simulink model "Rearranged_With_Subsystems"  (R2022b)
settings: Solver=ode15s  StartTime=0.0  StopTime=400  RelTol=1e-3
InitFcn:
  | ManipulatorSetup
  | init_quad_new_leg_raibert_strategy_v2
values from neighbouring files (symbols this model uses):
  body = 'obstacle'+string(i)    [GUIWithNavigation.m]    (also in RunModel.m)
  endx = 18    [EnvironmentData.mat]    (also in Practice data.mat = 15)
  endy = 18    [EnvironmentData.mat]    (also in Practice data.mat = 14)
  floorl = 20    [EnvironmentData.mat]    (also in GUIWithNavigation.m; Practice data.mat; RunModel.m)
  floorw = 20    [EnvironmentData.mat]    (also in GUIWithNavigation.m; Practice data.mat; RunModel.m)
  planner = plannerRRTStar(ss,stateValidator)    [GUIWithNavigation.m]    (also in RunModel.m)
  startx = 3    [EnvironmentData.mat]    (also in Practice data.mat = 2)
  starty = 3    [EnvironmentData.mat]    (also in Practice data.mat = 2)
  tar1Len = 10    [EnvironmentData.mat]    (also in GUIWithNavigation.m = length(target1); Practice data.mat = 13; RunModel.m = length(target1))
  target = [3 4.99844642156 6.95141646815 8.78790598722 9.67257563911 9.70990834754 10.5092252376 9.30187214417 9.05327436398 9.4 9.4 10.8486938703 ... (44 elements, 22x2)]    [EnvironmentData.mat]    (also in GUIWithNavigation.m = cat(1,target1,target2); Practice data.mat = [2 3.44057581018 5.07942513831 5.42542290116 7.21306818311 8; RunModel.m = cat(1,target1,target2))
  tarLen = 22    [EnvironmentData.mat]    (also in RunModel.m = length(target))
undefined symbols (not defined in the file or in its folder): closeFingers, ctrl, Extr_Data_LinkEndHole, grabObjectAngles, grabObjectAngles2, ground, holdFingers, homeAngles, inverseKinematicWeights, l1, l2, m1, m2, openFingers, readyAngles, X, Y, Z
libraries: sm_lib x459, nesl_utility x134, slpidlib x31, fl_ps_legacy_lib x6, robotmaniplib x6, simulink x5, fl_lib x5, Contact_Forces_Lib x4, Parts_Lib x4, sharedtransform x2, dspstat3 x1
(part 1 of 16)
settings Model: Creator=biorobotics  LastModifiedBy=uos
settings SolverCC: ZeroCrossAlgorithm=Adaptive  AlgebraicLoopSolver=TrustRegion
settings DataIOCC: ReturnWorkspaceOutputs=off
settings DebuggingCC: IgnoredZcDiagnostic=none  UnconnectedInputMsg=warning  UnconnectedOutputMsg=warning  UnconnectedLineMsg=warning  SFMachineParentedDataDiag=warning  ArithmeticOperatorsInVariantConditions=warning
settings ModelReferenceCC: EnableRefExpFcnMdlSchedulingChecks=on
settings SFSimCC: SimUseLocalCustomCode=off  CustomCodeUndefinedFunction=UseInterfaceOnly
settings RTWCC: RTWUseLocalCustomCode=off
settings DiagnosticsConfigSet: SimMechanicsRigidlyBoundBlock=none

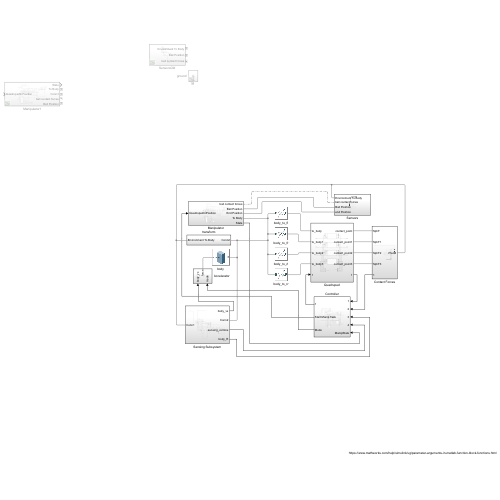
[thumbnail: Simulink's stored preview of the top-level diagram]
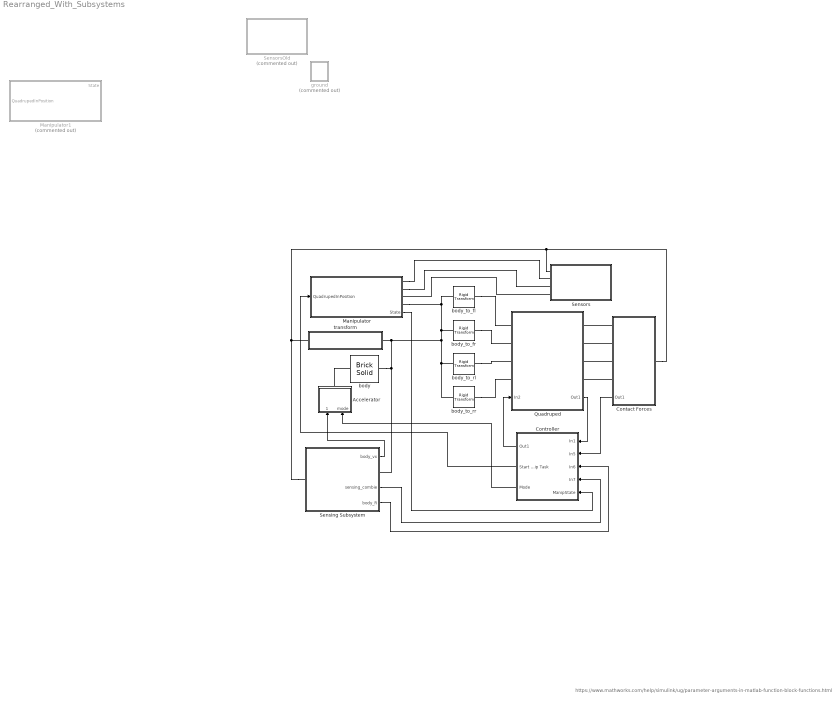
== system Rearranged_With_Subsystems ==
  note: https://www.mathworks.com/help/simulink/ug/parameter-arguments-in-matlab-function-block-functions.html
  Accelerator : Subsystem
      settings: PortSchema="{\"entries\":[{\"content\":{\"sides\":[{\"content\":{\"connectorIds\":[]},\"type\":\"ConnectorPlacement.EquallySpacedRectSide\",\"uuid\":\"3b8f4fb7-757d-44b0-8c84-ca404449afa6\"},{\"content\":{\"connectorIds\":[],\"side\":\"RIGHT\"},\"type\":\"ConnectorPlacement.EquallySpacedRectSide\",\"uuid\":\"4616ca68-8bb0-4699-a428-07415450d0e5\"},{\"content\":{\"connectorIds\":[\"LConn1\"],\"side\":\"TOP\"},\"type\":\"ConnectorPlacement.EquallySpacedRectSide\",\"uuid\":\"645a5e81-e5eb-476d-aa61-d9d757a3e189\"},{\"content\":{\"connectorIds\":[\"In1\",\"In2\"],\"side\":\"BOTTOM\"},\"type\":\"ConnectorPlacement.EquallySpacedRectSide\",\"uuid\":\"cfb89a5a-1661-4756-b538-cb5bbef02c9e\"}]},\"type\":\"ConnectorPlacement.EquallySpacedConnector\",\"uuid\":\"e64cce85-18e1-40ef-8b4c-1f7664925565\"}],\"packageUris\":[\"http://schema.mathworks.com/mf0/Connector/R2020b\"],\"version\":\"1.0\"}"
  Contact Forces : Subsystem
      settings: PortSchema="{\"entries\":[{\"content\":{\"sides\":[{\"content\":{\"connectorIds\":[\"LConn1\"]},\"type\":\"ConnectorPlacement.EquallySpacedRectSide\",\"uuid\":\"d9e77396-55f4-49e5-9c59-62df65a9aa33\"},{\"content\":{\"connectorIds\":[\"RConn1\",\"RConn2\",\"RConn3\",\"RConn4\",\"Out1\"],\"side\":\"RIGHT\"},\"type\":\"ConnectorPlacement.EquallySpacedRectSide\",\"uuid\":\"d655d73a-1d80-4dc0-89ee-c033d671b0c2\"},{\"content\":{\"connectorIds\":[],\"side\":\"TOP\"},\"type\":\"ConnectorPlacement.EquallySpacedRectSide\",\"uuid\":\"dc54e94d-e523-4784-8fd3-8e1e99781185\"},{\"content\":{\"connectorIds\":[],\"side\":\"BOTTOM\"},\"type\":\"ConnectorPlacement.EquallySpacedRectSide\",\"uuid\":\"f3bba4af-9235-4cb2-90c5-839fa8331c16\"}]},\"type\":\"ConnectorPlacement.EquallySpacedConnector\",\"uuid\":\"27dcd2a5-23bc-405e-9f4b-2eee189b7bee\"}],\"packageUris\":[\"http://schema.mathworks.com/mf0/Connector/R2020b\"],\"version\":\"1.0\"}"
  Controller : Subsystem
  Manipulator : Subsystem
      settings: PortSchema="{\"entries\":[{\"content\":{\"sides\":[{\"content\":{\"connectorIds\":[\"In1\"]},\"type\":\"ConnectorPlacement.EquallySpacedRectSide\",\"uuid\":\"ff2767ab-448c-4c0d-a9a4-8f0f2a440df5\"},{\"content\":{\"connectorIds\":[\"RConn1\",\"RConn2\",\"RConn3\",\"RConn4\",\"Out1\"],\"side\":\"RIGHT\"},\"type\":\"ConnectorPlacement.EquallySpacedRectSide\",\"uuid\":\"93606e9f-72dd-49b1-b6cf-e4d0c20d1a1a\"},{\"content\":{\"connectorIds\":[],\"side\":\"TOP\"},\"type\":\"ConnectorPlacement.EquallySpacedRectSide\",\"uuid\":\"db3624f7-6a1f-43d3-93ac-44b301eed69d\"}]},\"type\":\"ConnectorPlacement.EquallySpacedConnector\",\"uuid\":\"db27b8b3-f381-4b8d-9dee-3bd6b54b8be1\"}],\"packageUris\":[\"http://schema.mathworks.com/mf0/Connector/R2020b\"],\"version\":\"1.0\"}"
  Manipulator1 : Subsystem  Commented=on
  Quadruped : Subsystem
      settings: PortSchema="{\"entries\":[{\"content\":{\"sides\":[{\"content\":{\"connectorIds\":[\"LConn1\",\"LConn2\",\"LConn3\",\"LConn4\",\"In1\"]},\"type\":\"ConnectorPlacement.EquallySpacedRectSide\",\"uuid\":\"2b490502-7c0f-46f9-b6ce-17355d87bc82\"},{\"content\":{\"connectorIds\":[\"RConn1\",\"RConn2\",\"RConn3\",\"RConn4\",\"Out1\"],\"side\":\"RIGHT\"},\"type\":\"ConnectorPlacement.EquallySpacedRectSide\",\"uuid\":\"dcbb9991-2202-44f3-91f9-18bd7c5b50b3\"},{\"content\":{\"connectorIds\":[],\"side\":\"TOP\"},\"type\":\"ConnectorPlacement.EquallySpacedRectSide\",\"uuid\":\"5cc15507-c434-473a-bef2-323e772bf8f9\"}]},\"type\":\"ConnectorPlacement.EquallySpacedConnector\",\"uuid\":\"8c4551e2-5a1d-42e3-907a-2af9d6bfb3ed\"}],\"packageUris\":[\"http://schema.mathworks.com/mf0/Connector/R2020b\"],\"version\":\"1.0\"}"
  "Sensing Subsystem " : Subsystem
      settings: PortSchema="{\"entries\":[{\"content\":{\"sides\":[{\"content\":{\"connectorIds\":[\"LConn1\"]},\"type\":\"ConnectorPlacement.EquallySpacedRectSide\",\"uuid\":\"998221ad-fab7-44d6-86a8-33fec3ebf2d5\"},{\"content\":{\"connectorIds\":[\"Out1\",\"RConn1\",\"Out2\",\"Out3\"],\"side\":\"RIGHT\"},\"type\":\"ConnectorPlacement.EquallySpacedRectSide\",\"uuid\":\"413d99db-2567-4cd5-a930-0d9916e7d919\"},{\"content\":{\"connectorIds\":[],\"side\":\"TOP\"},\"type\":\"ConnectorPlacement.EquallySpacedRectSide\",\"uuid\":\"948855a1-4bad-45fb-bb01-4a3cbeb58f0f\"}]},\"type\":\"ConnectorPlacement.EquallySpacedConnector\",\"uuid\":\"705e2a16-9022-494f-aa05-78e7d130aa9c\"}],\"packageUris\":[\"http://schema.mathworks.com/mf0/Connector/R2020b\"],\"version\":\"1.0\"}"
  Sensors : Subsystem
  SensorsOld : Subsystem  Commented=on
  body : sm_lib/Body Elements/Brick Solid  GraphicAmbientColor=[0.15 0.15 0.15 1.0]  BasedOnType=Density  BrickDimensions=[body.x_length body.y_length body.z_length]  BrickDimensionUnits=m  CenterOfMass=[0 0 0]  CenterOfMassUnits=m  GraphicDiffuseColor=[164 184 200]/255  Density=600  DensityUnits=kg/(m^3)  DoExposeReferenceFrame=on  GraphicEmissiveColor=[0.0 0.0 0.0 1.0]  ExportEntireGeometry=off  SerializedFrames=<Frames><Frame><Id>Frame2</Id><Value><Name>force</Name><Origin><Source>CenterOfMassFrame</Source><FeatureName></FeatureName></Origin><PrimaryAxis><DefinedDirection>+Z</DefinedDirection><Source>ReferenceFrame</Source><SourceDirection>+Z</SourceDirection><FeatureName></FeatureName></PrimaryAxis><SecondaryAxis><DefinedDirection>+X</DefinedDirection><Source>ReferenceFrame</Source><SourceDirection>+X</SourceDirection><FeatureName></FeatureName></SecondaryAxis></Value></Frame></Frames>  MarkerShape=Sphere  MarkerSize=10  GraphicType=FromGeometry  InertiaType=CalculateFromGeometry  Mass=8.6  MassUnits=kg  MomentsOfInertia=[1 1 1]  MomentsOfInertiaUnits=kg*m^2  GraphicOpacity=1.0  ProductsOfInertia=[0 0 0]  ProductsOfInertiaUnits=kg*m^2  GraphicShininess=75  GraphicSpecularColor=[0.5 0.5 0.5 1.0]  GraphicVisPropType=SimpleVisualProperties
  body_to_fl : sm_lib/Frames and Transforms/Rigid Transform  TranslationMethod=Cartesian  TranslationStandardOffset=0  TranslationLengthUnit=m  TranslationStandardAxis=+Z  TranslationCartesianOffset=[body.shoulder_distance body.y_length/2+body.shoulder_size/2 0]  TranslationROffset=0  TranslationROffsetUnits=m  TranslationZOffset=0  TranslationZOffsetUnits=m  TranslationThetaOffset=0  TranslationThetaOffsetUnits=deg  RotationMethod=AlignedAxes  RotationAngleUnits=deg  RotationStandardAxis=+Z  RotationAngle=0.0  RotationArbitraryAxis=[0 0 1]  FollAlignAxisA=+Z  BaseAlignAxisA=+X  FollAlignAxisB=+X  BaseAlignAxisB=-Z  RotationSequenceAxes=FollowerAxes  RotationSequence=XYX  RotationSequenceAngles=[0 0 0]  RotationSequenceAnglesUnits=deg  RotationMatrix=[1 0 0; 0 1 0; 0 0 1]  Quaternion=[1 0 0 0]
  body_to_fr : sm_lib/Frames and Transforms/Rigid Transform  TranslationMethod=Cartesian  TranslationStandardOffset=0  TranslationLengthUnit=m  TranslationStandardAxis=+Z  TranslationCartesianOffset=[body.shoulder_distance -body.y_length/2-body.shoulder_size/2 0]  TranslationROffset=0  TranslationROffsetUnits=m  TranslationZOffset=0  TranslationZOffsetUnits=m  TranslationThetaOffset=0  TranslationThetaOffsetUnits=deg  RotationMethod=AlignedAxes  RotationAngleUnits=deg  RotationStandardAxis=+Z  RotationAngle=0.0  RotationArbitraryAxis=[0 0 1]  FollAlignAxisA=+Z  BaseAlignAxisA=+X  FollAlignAxisB=+X  BaseAlignAxisB=-Z  RotationSequenceAxes=FollowerAxes  RotationSequence=XYX  RotationSequenceAngles=[0 0 0]  RotationSequenceAnglesUnits=deg  RotationMatrix=[1 0 0; 0 1 0; 0 0 1]  Quaternion=[1 0 0 0]
  body_to_rl : sm_lib/Frames and Transforms/Rigid Transform  TranslationMethod=Cartesian  TranslationStandardOffset=0  TranslationLengthUnit=m  TranslationStandardAxis=+Z  TranslationCartesianOffset=[-body.shoulder_distance body.y_length/2+body.shoulder_size/2 0]  TranslationROffset=0  TranslationROffsetUnits=m  TranslationZOffset=0  TranslationZOffsetUnits=m  TranslationThetaOffset=0  TranslationThetaOffsetUnits=deg  RotationMethod=AlignedAxes  RotationAngleUnits=deg  RotationStandardAxis=+Z  RotationAngle=0.0  RotationArbitraryAxis=[0 0 1]  FollAlignAxisA=+Z  BaseAlignAxisA=+X  FollAlignAxisB=+X  BaseAlignAxisB=-Z  RotationSequenceAxes=FollowerAxes  RotationSequence=XYX  RotationSequenceAngles=[0 0 0]  RotationSequenceAnglesUnits=deg  RotationMatrix=[1 0 0; 0 1 0; 0 0 1]  Quaternion=[1 0 0 0]
  body_to_rr : sm_lib/Frames and Transforms/Rigid Transform  TranslationMethod=Cartesian  TranslationStandardOffset=0  TranslationLengthUnit=m  TranslationStandardAxis=+Z  TranslationCartesianOffset=[-body.shoulder_distance -body.y_length/2-body.shoulder_size/2 0]  TranslationROffset=0  TranslationROffsetUnits=m  TranslationZOffset=0  TranslationZOffsetUnits=m  TranslationThetaOffset=0  TranslationThetaOffsetUnits=deg  RotationMethod=AlignedAxes  RotationAngleUnits=deg  RotationStandardAxis=+Z  RotationAngle=0.0  RotationArbitraryAxis=[0 0 1]  FollAlignAxisA=+Z  BaseAlignAxisA=+X  FollAlignAxisB=+X  BaseAlignAxisB=-Z  RotationSequenceAxes=FollowerAxes  RotationSequence=XYX  RotationSequenceAngles=[0 0 0]  RotationSequenceAnglesUnits=deg  RotationMatrix=[1 0 0; 0 1 0; 0 0 1]  Quaternion=[1 0 0 0]
  ground : Subsystem  Commented=on
  transform : Subsystem
  wires:
  "Sensing Subsystem "/3(body_R) -> Controller/3(In6)
  "Sensing Subsystem "/2(sensing_combie) -> Controller/4(In7)
  Manipulator/1(State) -> Controller/5(ManipState)
  Controller/2(Start Manip Task) -> Manipulator/1(QuadrupedInPosition)
  Controller/3(Mode) -> Accelerator/2(mode)
  "Sensing Subsystem "/1(body_vx) -> Accelerator/1(body_vx)
  Quadruped/1(Out1) -> Controller/1(In1)
  Contact Forces/1(Out1) -> Controller/2(In5)
  Controller/1(Out1) -> Quadruped/1(In2)
  connections:
  Manipulator/RConn4 -- body_to_fl/LConn1 -- body_to_rr/LConn1 -- body_to_rl/LConn1 -- body/RConn1 -- "Sensing Subsystem "/RConn1 -- transform/LConn1 -- body_to_fr/LConn1
  Manipulator/RConn1 -- Sensors/RConn2
  Manipulator/RConn2 -- Sensors/RConn3
  Sensors/RConn4 -- Manipulator/RConn3
  Accelerator/LConn1 -- body/LConn1
  body_to_fl/RConn1 -- Quadruped/LConn1
  body_to_fr/RConn1 -- Quadruped/LConn2
  body_to_rl/RConn1 -- Quadruped/LConn3
  body_to_rr/RConn1 -- Quadruped/LConn4
  "Sensing Subsystem "/LConn1 -- Contact Forces/LConn1 -- Sensors/RConn1 -- transform/RConn1
  Contact Forces/RConn1 -- Quadruped/RConn1
  Contact Forces/RConn2 -- Quadruped/RConn2
  Contact Forces/RConn3 -- Quadruped/RConn3
  Contact Forces/RConn4 -- Quadruped/RConn4

== system Rearranged_With_Subsystems/Accelerator ==
  body_vx : Inport
  mode : Inport  Port=2
  Constant : Constant  Value=100
  Constant1 : Constant  Value=0
  Constant2 : Constant  Value=2
  Constant3 : Constant  Value=0.5
  External Force and Torque : sm_lib/Forces and Torques/External Force and Torque  ForceResolutionFrame=AttachedFrame  EnableForceX=on  EnableForceY=off  EnableForceZ=off  EnableForce=off  TorqueResolutionFrame=AttachedFrame  EnableTorqueX=off  EnableTorqueY=off  EnableTorqueZ=off  EnableTorque=off
  Logical Operator : Logic  AllPortsSameDT=off  OutDataTypeStr=boolean
  Moving Average : dspstat3/Moving Average  Method=Sliding window  ForgettingFactorPort=off  SpecifyWindowLength=on  WindowLength=10  OverlapLength=9  AllowArbitraryInputLength=off  ForgettingFactor=0.9  SimulateUsing=Code generation
  Relational Operator : RelationalOperator  Operator=<  OutDataTypeStr=boolean  RndMeth=Simplest  InputSameDT=off
  Relational Operator1 : RelationalOperator  Operator=<  OutDataTypeStr=boolean  RndMeth=Simplest  InputSameDT=off
  Simulink-PS Converter : nesl_utility/Simulink-PS Converter  PhysicalDomain=network_engine_domain  SubClassName=ps_input  LeftPortType=input  RightPortType=output  PseudoPeriodic=off  Frequencies=[]  NoiseDistribution=none  NoiseParameters=[]  Unit=1  AffineConversion=off  FilteringAndDerivatives=provide  SimscapeFilterOrder=1  InputFilterTimeConstant=0.001  UdotUserProvided=0
  Switch : Switch  Criteria=u2 > Threshold  SaturateOnIntegerOverflow=off  InputSameDT=off
  force : PMIOPort  Side=Left
  wires:
  Switch/1 -> Simulink-PS Converter/1
  Constant/1 -> Switch/1
  Relational Operator/1 -> Logical Operator/1
  Relational Operator1/1 -> Logical Operator/2
  Logical Operator/1 -> Switch/2
  Moving Average/1 -> Relational Operator1/1
  Constant2/1 -> Relational Operator/2
  Constant3/1 -> Relational Operator1/2
  mode/1 -> Relational Operator/1
  body_vx/1 -> Moving Average/1
  Constant1/1 -> Switch/3
  connections:
  force/RConn1 -- External Force and Torque/RConn1
  External Force and Torque/LConn1 -- Simulink-PS Converter/RConn1

== system Rearranged_With_Subsystems/Contact Forces ==
  Bus Creator : BusCreator  Inputs=4
  Contact_fl : Subsystem
  Contact_fr : Subsystem
  Contact_rl : Subsystem
  Contact_rr : Subsystem
  PlanB : PMIOPort  Side=Left
  SphF : PMIOPort  Port=2  Side=Right
  SphF1 : PMIOPort  Port=3  Side=Right
  SphF2 : PMIOPort  Port=4  Side=Right
  SphF3 : PMIOPort  Port=5  Side=Right
  Out1 : Outport
  wires:
  Contact_fl/1(state) -> Bus Creator/1
  Contact_fr/1(state) -> Bus Creator/2
  Contact_rl/1(state) -> Bus Creator/3
  Contact_rr/1(state) -> Bus Creator/4
  Bus Creator/1 -> Out1/1
  connections:
  Contact_fr/LConn1 -- PlanB/RConn1 -- Contact_fl/LConn1 -- Contact_rr/LConn1 -- Contact_rl/LConn1
  Contact_rl/RConn1 -- SphF2/RConn1
  Contact_fl/RConn1 -- SphF/RConn1
  Contact_fr/RConn1 -- SphF1/RConn1
  Contact_rr/RConn1 -- SphF3/RConn1

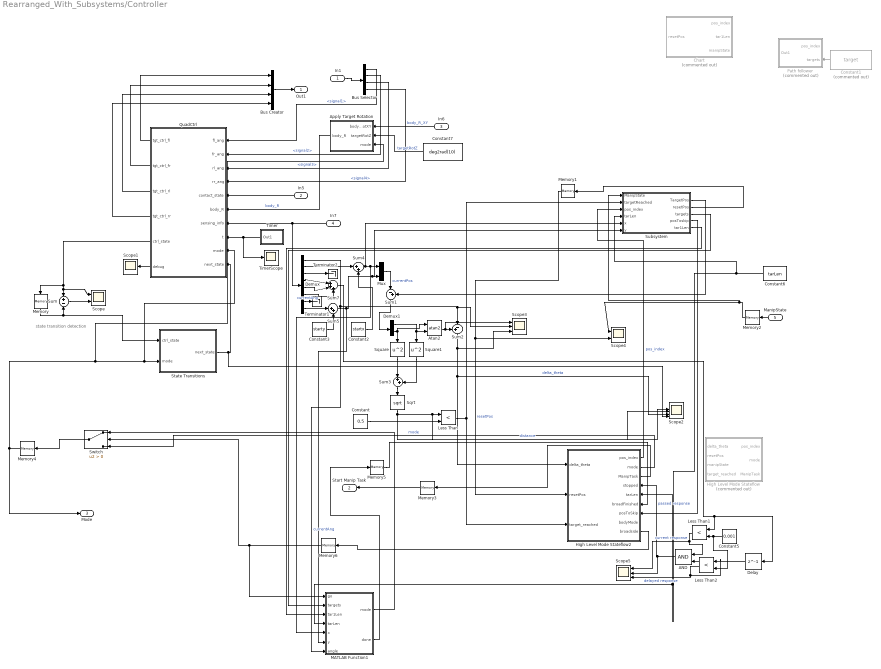
== system Rearranged_With_Subsystems/Controller ==
  note: state transition detection
  In1 : Inport
  In5 : Inport  Port=2
  In6 : Inport  Port=3
  In7 : Inport  Port=4
  ManipState : Inport  Port=5
  AND : Logic  IconShape=distinctive  AllPortsSameDT=off  OutDataTypeStr=boolean
  Apply Target Rotation : Subsystem
  Atan2 : Trigonometry  Operator=atan2
  Bus Creator : BusCreator  Inputs=4
  Bus Selector : BusSelector  OutputSignals=signal1,signal2,signal3,signal4
  Chart : Stateflow chart  Commented=on  TreatAsAtomicUnit=on
  Constant : Constant  Value=0.5
  Constant1 : Constant  Commented=on  Value=target
  Constant2 : Constant  Value=startx
  Constant3 : Constant  Value=starty
  Constant5 : Constant  Value=0.001
  Constant6 : Constant  Value=tarLen
  Constant7 : Constant  Value=deg2rad(10)
  Delay : Delay  DelayLength=1
  Demux : Demux  Outputs=8
  Demux1 : Demux  Outputs=2
  High Level Mode Stateflow : Stateflow chart  Commented=on  TreatAsAtomicUnit=on
      settings: PortSchema="{\"entries\":[{\"content\":{\"sides\":[{\"content\":{\"connectorIds\":[\"In2\",\"In3\",\"In4\",\"In1\"]},\"type\":\"ConnectorPlacement.EquallySpacedRectSide\",\"uuid\":\"54635eaa-af22-4c07-946c-8b3764ca4079\"},{\"content\":{\"connectorIds\":[\"Out1\",\"Out2\",\"Out3\"],\"side\":\"RIGHT\"},\"type\":\"ConnectorPlacement.EquallySpacedRectSide\",\"uuid\":\"b8ca9e50-c21e-481d-aebe-d3447dd5b6ec\"},{\"content\":{\"connectorIds\":[],\"side\":\"TOP\"},\"type\":\"ConnectorPlacement.EquallySpacedRectSide\",\"uuid\":\"aa364018-0c1f-4137-8fa7-722b902e07a1\"}]},\"type\":\"ConnectorPlacement.EquallySpacedConnector\",\"uuid\":\"b87c06e7-bef4-4368-b066-66035be64295\"}],\"packageUris\":[\"http://schema.mathworks.com/mf0/Connector/R2020b\"],\"version\":\"1.0\"}"
  High Level Mode Stateflow2 : Stateflow chart  TreatAsAtomicUnit=on
      settings: PortSchema="{\"entries\":[{\"content\":{\"sides\":[{\"content\":{\"connectorIds\":[\"In2\",\"In3\",\"In1\"]},\"type\":\"ConnectorPlacement.EquallySpacedRectSide\",\"uuid\":\"54635eaa-af22-4c07-946c-8b3764ca4079\"},{\"content\":{\"connectorIds\":[\"Out1\",\"Out2\",\"Out3\",\"In4\",\"In5\",\"In6\",\"In7\",\"Out4\",\"Out5\"],\"side\":\"RIGHT\"},\"type\":\"ConnectorPlacement.EquallySpacedRectSide\",\"uuid\":\"b8ca9e50-c21e-481d-aebe-d3447dd5b6ec\"},{\"content\":{\"connectorIds\":[],\"side\":\"TOP\"},\"type\":\"ConnectorPlacement.EquallySpacedRectSide\",\"uuid\":\"aa364018-0c1f-4137-8fa7-722b902e07a1\"}]},\"type\":\"ConnectorPlacement.EquallySpacedConnector\",\"uuid\":\"b87c06e7-bef4-4368-b066-66035be64295\"}],\"packageUris\":[\"http://schema.mathworks.com/mf0/Connector/R2020b\"],\"version\":\"1.0\"}"
  Less Than : RelationalOperator  Operator=<  OutDataTypeStr=boolean  RndMeth=Simplest  InputSameDT=off
  Less Than1 : RelationalOperator  Operator=<  OutDataTypeStr=boolean  RndMeth=Simplest  InputSameDT=off
  Less Than2 : RelationalOperator  Operator=<  OutDataTypeStr=boolean  RndMeth=Simplest  InputSameDT=off
  MATLAB Function1 : MATLAB Function  TreatAsAtomicUnit=on
  Memory{,1..6} (7 alike) : Memory
  Mux : Mux  Inputs=2
  Path follower : Subsystem  Commented=on  TreatAsAtomicUnit=on
  QuadCtrl : MATLAB Function  TreatAsAtomicUnit=on  SystemSampleTime=0.0025
  Scope : Scope  NumInputPorts=2
  Scope1 : Scope
  Scope2 : Scope  NumInputPorts=6
  Scope3 : Scope  NumInputPorts=3
  Scope4 : Scope  NumInputPorts=2
  Scope5 : Scope  NumInputPorts=3
  Sqrt : Sqrt
  Square : Math  Operator=square
  Square1 : Math  Operator=square
  State Transitions : Stateflow chart  TreatAsAtomicUnit=on
  Subsystem : Subsystem
  Sum : Sum  Inputs=+-
  Sum1 : Sum  Inputs=|-+
  Sum2 : Sum  Inputs=+-|
  Sum3 : Sum  Inputs=|++
  Sum4 : Sum  Inputs=|++
  Sum5 : Sum  Inputs=|++
  Sum7 : Sum  Inputs=|+++
  Switch : Switch  Criteria=u2 > Threshold  SaturateOnIntegerOverflow=off  InputSameDT=off
  Terminator1 : Terminator
  Terminator2 : Terminator
  Timer : Subsystem
  TimerScope : Scope
  Out1 : Outport  VectorParamsAs1DForOutWhenUnconnected=off
  Start Manip Task : Outport  Port=2  VectorParamsAs1DForOutWhenUnconnected=off
  Mode : Outport  Port=3
  wires:
  In7/1 -> Demux/1, QuadCtrl/7(sensing_info)
  Timer/1(Out1) -> TimerScope/1, QuadCtrl/8(t)
  In5/1 -> QuadCtrl/5(contact_state)
  QuadCtrl/3(tgt_ctrl_rl) -> Bus Creator/3
  QuadCtrl/2(tgt_ctrl_fr) -> Bus Creator/2
  QuadCtrl/4(tgt_ctrl_rr) -> Bus Creator/4
  QuadCtrl/5(ctrl_state) -> Scope/1, Sum/1, Memory/1
  Memory/1 -> State Transitions/1(ctrl_state), Sum/2
  Sum/1 -> Scope/2
  QuadCtrl/6(debug) -> Scope1/1
  Less Than/1 -> Subsystem/2(targetReached), High Level Mode Stateflow2/1(target_reached)
  Sum2/1 -> High Level Mode Stateflow2/2(delta_theta), Scope2/5, Scope3/3  "delta_theta"
  Demux/3 -> Terminator2/1
  Demux/4 -> Sum7/1
  Demux/5 -> Sum7/2
  Mux/1 -> Sum1/1  "currentPos"
  Sum1/1 -> Demux1/1
  Demux1/1 -> Atan2/2, Square1/1
  Demux1/2 -> Atan2/1, Square/1
  Atan2/1 -> Scope3/1, Sum2/1
  Sum3/1 -> Sqrt/1
  Square1/1 -> Sum3/2
  Square/1 -> Sum3/1
  Sqrt/1 -> Scope2/3, Scope2/4, Less Than/1  "distance"
  Constant/1 -> Less Than/2
  State Transitions/1(next_state) -> QuadCtrl/10(next_state), Scope2/6
  Demux/2 -> Sum4/1
  Demux/8 -> Sum5/1
  Constant2/1 -> Sum4/2
  Constant3/1 -> Sum5/2
  Sum4/1 -> Subsystem/5(x), MATLAB Function1/5(x), Mux/1
  Sum5/1 -> MATLAB Function1/6(y), Subsystem/6(y), Mux/2
  Demux/1 -> MATLAB Function1/7(angle), Scope3/2, Sum2/2  "currentAng"
  Constant6/1 -> Subsystem/4(tarLen), MATLAB Function1/4(tarLen), High Level Mode Stateflow2/5(tarLen)
  Memory1/1 -> High Level Mode Stateflow2/3(resetPos), Scope4/2  "resetPos"
  ManipState/1 -> Memory2/1
  Memory2/1 -> Subsystem/1(ManipState), Scope4/1
  Memory3/1 -> Start Manip Task/1
  Constant1/1 -> Path follower/2(targets)
  Demux/6 -> Sum7/3
  Constant5/1 -> Less Than2/2, Less Than1/2
  Sum7/1 -> Delay/1, Less Than1/1
  MATLAB Function1/2(done) -> Memory5/1
  MATLAB Function1/1(mode) -> Switch/1
  Memory4/1 -> Apply Target Rotation/3(mode), State Transitions/2(mode), QuadCtrl/9(mode), Mode/1
  Memory6/1 -> MATLAB Function1/1(go), Switch/2
  Switch/1 -> Memory4/1
  Constant7/1 -> Apply Target Rotation/2(targetRotZ)  "targetRotZ"
  In6/1 -> Apply Target Rotation/1(body_RotXY)  "body_R_XY"
  Apply Target Rotation/1(body_R) -> QuadCtrl/6(body_R)  "body_R"
  Demux/7 -> Terminator1/1  "currentAng"
  Memory5/1 -> High Level Mode Stateflow2/6(broadFinished)
  High Level Mode Stateflow2/1(pos_index) -> Subsystem/3(pos_index)  "pos_index"
  High Level Mode Stateflow2/3(ManipTask) -> Memory3/1
  High Level Mode Stateflow2/5(broadside) -> Memory6/1
  High Level Mode Stateflow2/2(mode) -> Switch/3  "mode"
  Subsystem/1(TargetPos) -> Sum1/2
  Subsystem/2(resetPos) -> Memory1/1
  Subsystem/3(targets) -> MATLAB Function1/2(targets)
  Subsystem/5(tar1Len) -> MATLAB Function1/3(tar1Len)
  Subsystem/4(posToskip) -> High Level Mode Stateflow2/7(posToSkip)
  Delay/1 -> Less Than2/1
  Less Than1/1 -> AND/1, Scope5/1  "current response"
  Less Than2/1 -> AND/2, Scope5/3  "delayed response"
  AND/1 -> Scope5/2, High Level Mode Stateflow2/4(stopped)  "passed response"
  Bus Creator/1 -> Out1/1
  QuadCtrl/1(tgt_ctrl_fl) -> Bus Creator/1
  In1/1 -> Bus Selector/1
  Bus Selector/1 -> QuadCtrl/1(fl_ang)  "<signal1>"
  Bus Selector/2 -> QuadCtrl/2(fr_ang)  "<signal2>"
  Bus Selector/3 -> QuadCtrl/3(rl_ang)  "<signal3>"
  Bus Selector/4 -> QuadCtrl/4(rr_ang)  "<signal4>"
